simulink model "lab_6"  (R2015a)
settings: Solver=ode45  StartTime=0.0  StopTime=1  RelTol=1e-3
libraries: powerlib x13, powerlib_meascontrol x6
settings Model: Creator=DHARMIK  LastModifiedBy=DHARMIK

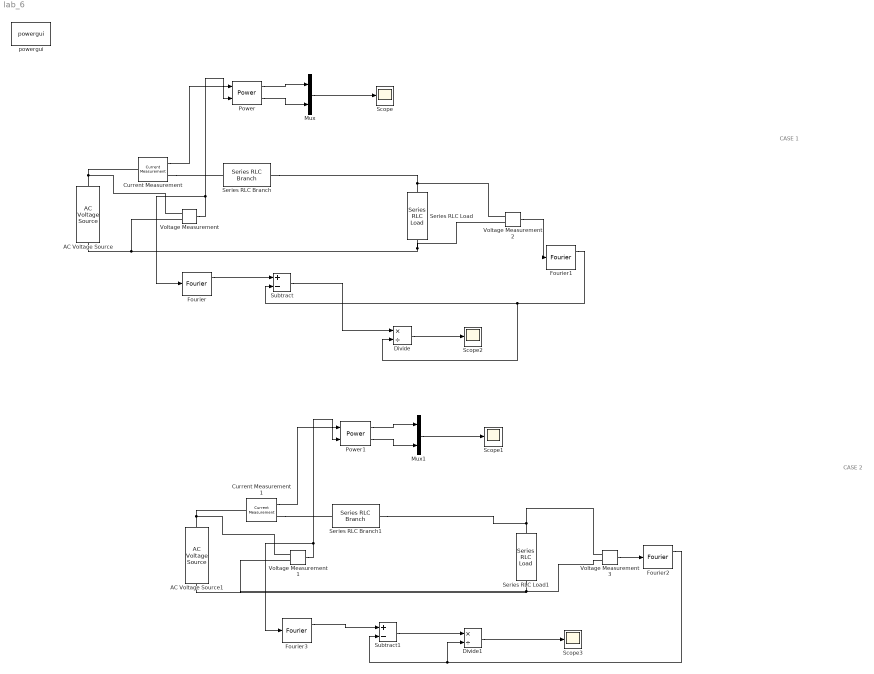
== system lab_6 ==
  note: CASE 2
  note: CASE 1
  AC Voltage Source : powerlib/Electrical Sources/AC Voltage Source  Amplitude=200998.5752  Phase=3.92  Frequency=50  SampleTime=0  Measurements=None
  AC Voltage Source1 : powerlib/Electrical Sources/AC Voltage Source  Amplitude=173945.608  Phase=7.9018  Frequency=50  SampleTime=0  Measurements=None
  Current Measurement : powerlib/Measurements/Current Measurement  PhasorSimulation=off  OutputType=Complex  PSBequivalent=0
  Current Measurement1 : powerlib/Measurements/Current Measurement  PhasorSimulation=off  OutputType=Complex  PSBequivalent=0
  Divide : Product  Inputs=*/
  Divide1 : Product  Inputs=*/
  Fourier{,1..3} (4 alike) : powerlib_meascontrol/Measurements/Fourier  Freq=60  n=1  InInit=[0, 0]  Ts=0
  Mux : Mux  Inputs=2
  Mux1 : Mux  Inputs=2
  Power : powerlib_meascontrol/Measurements/Power  Freq=50  Vinit=[1, 0]  Iinit=[1, 0]  Ts=0
  Power1 : powerlib_meascontrol/Measurements/Power  Freq=50  Vinit=[1, 0]  Iinit=[1, 0]  Ts=0
  Scope{,1..3} (4 alike) : Scope
      Scope settings: ShowLegends=on  YMin=-1e+08  YMax=1.2e+08
      Scope1 settings: ShowLegends=on  YMin=-1e+08  YMax=1.2e+08
      Scope2 settings: ShowLegends=on  YMin=-1e+08  YMax=1.2e+08  SaveName=ScopeData2
      Scope3 settings: ShowLegends=on  YMin=-1e+08  YMax=1.2e+08  SaveName=ScopeData3
  Series RLC Branch : powerlib/Elements/Series RLC Branch  LConnTagsString=__new0  RConnTagsString=__new0  BranchType=RL  Resistance=6  Inductance=52.923e-3  SetiL0=off  InitialCurrent=0  Capacitance=1e-6  Setx0=off  InitialVoltage=0  Measurements=None
  Series RLC Branch1 : powerlib/Elements/Series RLC Branch  LConnTagsString=__new0  RConnTagsString=__new0  BranchType=RL  Resistance=6  Inductance=52.923e-3  SetiL0=off  InitialCurrent=0  Capacitance=1e-6  Setx0=off  InitialVoltage=0  Measurements=None
  Series RLC Load : powerlib/Elements/Series RLC Load  LConnTagsString=a  RConnTagsString=__new0  NominalVoltage=1.2702e+05  NominalFrequency=50  ActivePower=101600000  InductivePower=76200000  CapacitivePower=0  Setx0=off  InitialVoltage=0  SetiL0=off  InitialCurrent=0  Measurements=None
  Series RLC Load1 : powerlib/Elements/Series RLC Load  LConnTagsString=a  RConnTagsString=__new0  NominalVoltage=1.2702e+05  NominalFrequency=50  ActivePower=101600000  InductivePower=0  CapacitivePower=76200000  Setx0=off  InitialVoltage=0  SetiL0=off  InitialCurrent=0  Measurements=None
  Subtract : Sum  Inputs=+-
  Subtract1 : Sum  Inputs=+-
  Voltage Measurement{,1..3} (4 alike) : powerlib/Measurements/Voltage Measurement  PhasorSimulation=off  OutputType=Complex  PSBequivalent=0
  powergui : powerlib/powergui  Priority=1  SimulationMode=Discrete  SolverType=Tustin/Backward Euler (TBE)  SampleTime=50e-6  frequency=60  SPID=off  DisableSnubberDevices=off  DisableRonSwitches=off  DisableVfSwitches=off  SwTol=0  DisplayEquations=off  Interpol=off  methode=off  Ts=100  FunctionMessages=off  echomessages=off  HookPort=off  EnableUseOfTLC=off  x0status=blocks  frequencyindice=50  Pbase=100e6  ErrMax=1e-4  Iterations=50  UnitsV=kV  UnitsW=MW  buscounter=0  RestoreLinks=warning  ResistiveCurrentMeasurement=off  Frange=[0:2:500]  Ylog=off  Xlog=on  ShowGrid=off  save=off  variable=ZData  structure=0  ZoomFFT=off  StartTime=0.0  cycles=1  DisplayStyle=1  fundamental=60  FreqAxis=off  MaxFrequency=1000  frequencyindicesteady=1  RmsSteady=1  display=off
  wires:
  Mux/1 -> Scope/1
  Voltage Measurement/1 -> Fourier/1, Power/1
  Current Measurement/1 -> Power/2
  Power/1 -> Mux/1
  Power/2 -> Mux/2
  Mux1/1 -> Scope1/1
  Voltage Measurement1/1 -> Fourier3/1, Power1/1
  Current Measurement1/1 -> Power1/2
  Power1/1 -> Mux1/1
  Power1/2 -> Mux1/2
  Voltage Measurement2/1 -> Fourier1/1
  Fourier/1 -> Subtract/1
  Fourier1/1 -> Divide/2, Subtract/2
  Subtract/1 -> Divide/1
  Divide/1 -> Scope2/1
  Voltage Measurement3/1 -> Fourier2/1
  Fourier3/1 -> Subtract1/1
  Fourier2/1 -> Divide1/2, Subtract1/2
  Subtract1/1 -> Divide1/1
  Divide1/1 -> Scope3/1
  connections:
  AC Voltage Source/LConn1 -- Voltage Measurement/LConn2 -- Voltage Measurement2/LConn2 -- Series RLC Load/LConn1
  Series RLC Branch/RConn1 -- Voltage Measurement2/LConn1 -- Series RLC Load/RConn1
  Current Measurement/RConn1 -- Series RLC Branch/LConn1
  AC Voltage Source/RConn1 -- Voltage Measurement/LConn1 -- Current Measurement/LConn1
  AC Voltage Source1/LConn1 -- Voltage Measurement1/LConn2 -- Voltage Measurement3/LConn2 -- Series RLC Load1/LConn1
  AC Voltage Source1/RConn1 -- Voltage Measurement1/LConn1 -- Current Measurement1/LConn1
  Current Measurement1/RConn1 -- Series RLC Branch1/LConn1
  Voltage Measurement3/LConn1 -- Series RLC Branch1/RConn1 -- Series RLC Load1/RConn1
